simulink model "Punto_9"  (R2022a)
settings: Solver=VariableStepAuto  StartTime=0.0  StopTime=10.0  RelTol=1e-3
undefined symbols (not defined in the file): A, B
settings Model: Creator=garzo  LastModifiedBy=garzo

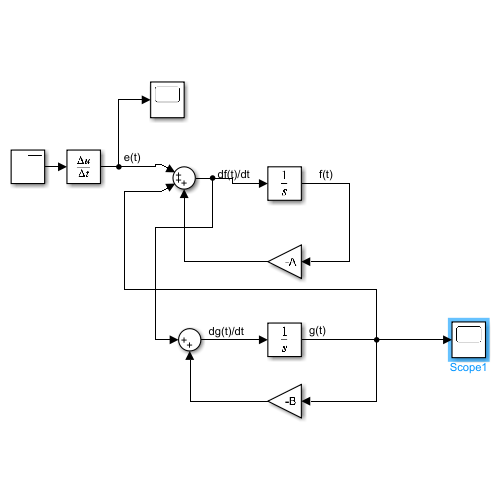
[thumbnail: Simulink's stored preview of the top-level diagram]
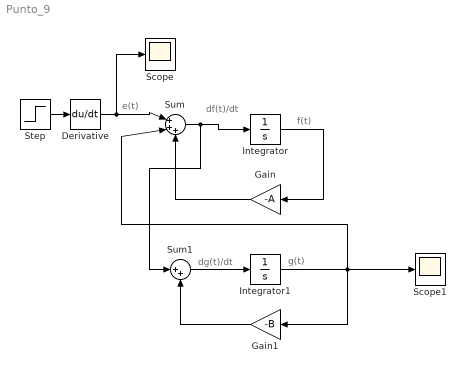
== system Punto_9 ==
  note: g(t)
  note: f(t)
  note: df(t)/dt
  note: e(t)
  note: dg(t)/dt
  Derivative : Derivative
  Gain : Gain  Gain=-A
  Gain1 : Gain  Gain=-B
  Integrator : Integrator
  Integrator1 : Integrator
  Scope : Scope
  Scope1 : Scope
  Step : Step  SampleTime=0
  Sum : Sum  Inputs=|+++
  Sum1 : Sum  Inputs=|++
  wires:
  Gain/1 -> Sum/3
  Integrator1/1 -> Sum/2, Scope1/1, Gain1/1
  Sum1/1 -> Integrator1/1
  Sum/1 -> Sum1/1, Integrator/1
  Gain1/1 -> Sum1/2
  Integrator/1 -> Gain/1
  Step/1 -> Derivative/1
  Derivative/1 -> Scope/1, Sum/1
